simulink model "storage_tester"  (R2024b)
settings: Solver=ode1  StartTime=0.0  StopTime=50  FixedStep=0.05  RelTol=1e-3
libraries: storage_lib x3
settings Model: Creator=marcv  LastModifiedBy=marcv
settings RTWCC: GPUComputeCapability=3.5

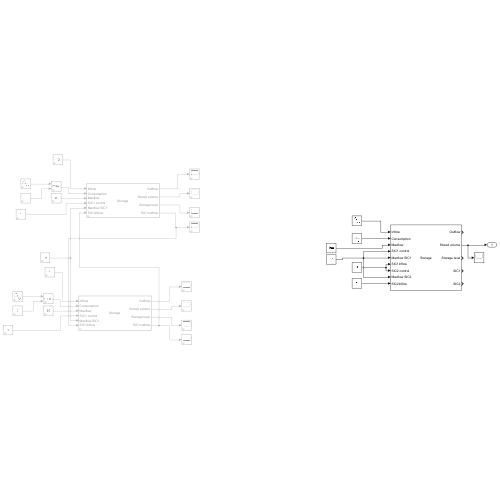
[thumbnail: Simulink's stored preview of the top-level diagram]
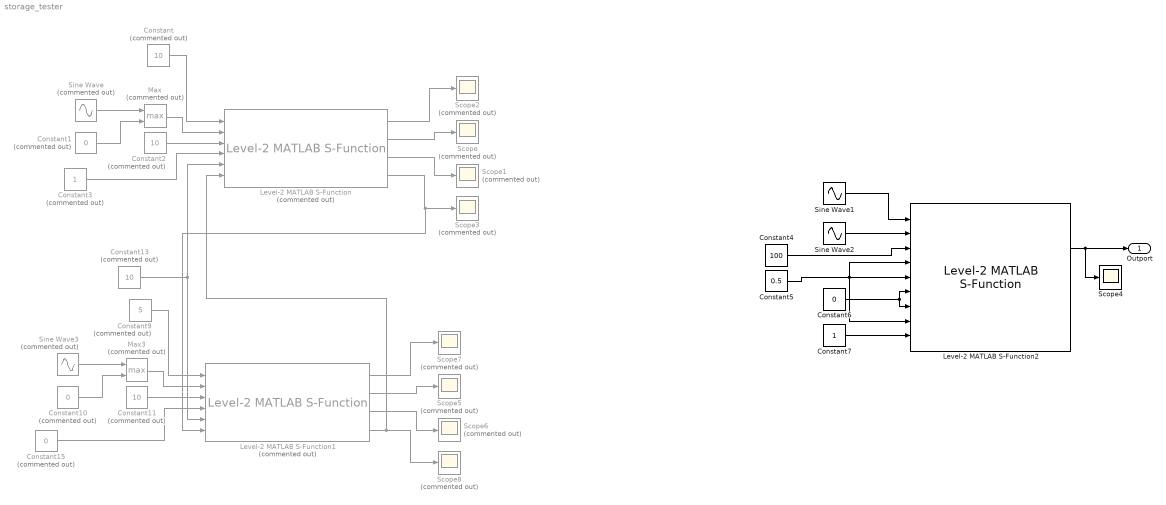
== system storage_tester ==
  Constant{,2,11,13} (4 alike) : Constant  Commented=on  Value=10
  Constant1 : Constant  Commented=on  Value=0
  Constant10 : Constant  Commented=on  Value=0
  Constant15 : Constant  Commented=on  Value=0
  Constant3 : Constant  Commented=on
  Constant4 : Constant  Value=100
  Constant5 : Constant  Value=0.5
  Constant6 : Constant  Value=0
  Constant7 : Constant
  Constant9 : Constant  Commented=on  Value=5
  Level-2 MATLAB S-Function : storage_lib/Level-2 MATLAB S-Function  Commented=on  Parameter1=500  Parameter2=0.2  Parameter3=1 interconnection
  Level-2 MATLAB S-Function1 : storage_lib/Level-2 MATLAB S-Function  Commented=on  Parameter1=500  Parameter2=0.2  Parameter3=1 interconnection
  Level-2 MATLAB S-Function2 : storage_lib/Level-2 MATLAB S-Function  Parameter1=20000  Parameter2=0.0005  Parameter3=2 interconnections
  Max : MinMax  Commented=on  Function=max  Inputs=2
  Max3 : MinMax  Commented=on  Function=max  Inputs=2
  Scope{,1..3,5..8} (8 alike) : Scope  Commented=on
  Scope4 : Scope
  Sine Wave : Sin  Commented=on  Amplitude=20  SampleTime=0
  Sine Wave1 : Sin  Amplitude=2  Bias=2  Frequency=1/5  SampleTime=0
  Sine Wave2 : Sin  Amplitude=2  Bias=2  SampleTime=0
  Sine Wave3 : Sin  Commented=on  Amplitude=20  SampleTime=0
  Outport : Outport
  wires:
  Constant/1 -> Level-2 MATLAB S-Function/1
  Level-2 MATLAB S-Function/1 -> Scope2/1
  Level-2 MATLAB S-Function/2 -> Scope/1
  Level-2 MATLAB S-Function/3 -> Scope1/1
  Max/1 -> Level-2 MATLAB S-Function/2
  Sine Wave/1 -> Max/1
  Constant1/1 -> Max/2
  Constant2/1 -> Level-2 MATLAB S-Function/3
  Constant13/1 -> Level-2 MATLAB S-Function1/5, Level-2 MATLAB S-Function/5
  Constant3/1 -> Level-2 MATLAB S-Function/4
  Level-2 MATLAB S-Function1/4 -> Level-2 MATLAB S-Function/6, Scope8/1
  Sine Wave3/1 -> Max3/1
  Max3/1 -> Level-2 MATLAB S-Function1/2
  Level-2 MATLAB S-Function/4 -> Level-2 MATLAB S-Function1/6, Scope3/1
  Level-2 MATLAB S-Function1/3 -> Scope6/1
  Constant11/1 -> Level-2 MATLAB S-Function1/3
  Constant9/1 -> Level-2 MATLAB S-Function1/1
  Constant10/1 -> Max3/2
  Level-2 MATLAB S-Function1/2 -> Scope5/1
  Level-2 MATLAB S-Function1/1 -> Scope7/1
  Constant15/1 -> Level-2 MATLAB S-Function1/4
  Sine Wave1/1 -> Level-2 MATLAB S-Function2/1
  Sine Wave2/1 -> Level-2 MATLAB S-Function2/2
  Constant4/1 -> Level-2 MATLAB S-Function2/3
  Constant5/1 -> Level-2 MATLAB S-Function2/8, Level-2 MATLAB S-Function2/5, Level-2 MATLAB S-Function2/4
  Constant6/1 -> Level-2 MATLAB S-Function2/6, Level-2 MATLAB S-Function2/7
  Constant7/1 -> Level-2 MATLAB S-Function2/9
  Level-2 MATLAB S-Function2/2 -> Outport/1, Scope4/1
